simulink model "Rail_SetPointCor"  (R2016b)
settings: configuration reference "CodeGenConfigSet" (kept outside this file)
values from neighbouring files (symbols this model uses):
  Rail_facSetPointAPSCor_CUR = Calibration.Parameter    [init_Rail_SetPointCor.m]    (also in init_Rail_SetPointCor_SIL.m = Simulink.Parameter)
  Rail_facSetPointAPSCor_CURX = Calibration.Parameter    [init_Rail_SetPointCor.m]    (also in init_Rail_SetPointCor_SIL.m = Simulink.Parameter)
  Rail_facSetPointATSCor_CUR = Calibration.Parameter    [init_Rail_SetPointCor.m]    (also in init_Rail_SetPointCor_SIL.m = Simulink.Parameter)
  Rail_facSetPointATSCor_CURX = Calibration.Parameter    [init_Rail_SetPointCor.m]    (also in init_Rail_SetPointCor_SIL.m = Simulink.Parameter)
  Rail_facSetPointETSCor_CUR = Calibration.Parameter    [init_Rail_SetPointCor.m]    (also in init_Rail_SetPointCor_SIL.m = Simulink.Parameter)
  Rail_facSetPointETSCor_CURX = Calibration.Parameter    [init_Rail_SetPointCor.m]    (also in init_Rail_SetPointCor_SIL.m = Simulink.Parameter)
  Rail_pSetPointAPSCor_MAP = Calibration.Parameter    [init_Rail_SetPointCor.m]    (also in init_Rail_SetPointCor_SIL.m = Simulink.Parameter)
  Rail_pSetPointAPSCor_MAPX = Calibration.Parameter    [init_Rail_SetPointCor.m]    (also in init_Rail_SetPointCor_SIL.m = Simulink.Parameter)
  Rail_pSetPointAPSCor_MAPY = Calibration.Parameter    [init_Rail_SetPointCor.m]    (also in init_Rail_SetPointCor_SIL.m = Simulink.Parameter)
  Rail_pSetPointATSCor_MAP = Calibration.Parameter    [init_Rail_SetPointCor.m]    (also in init_Rail_SetPointCor_SIL.m = Simulink.Parameter)
  Rail_pSetPointATSCor_MAPX = Calibration.Parameter    [init_Rail_SetPointCor.m]    (also in init_Rail_SetPointCor_SIL.m = Simulink.Parameter)
  Rail_pSetPointATSCor_MAPY = Calibration.Parameter    [init_Rail_SetPointCor.m]    (also in init_Rail_SetPointCor_SIL.m = Simulink.Parameter)
  Rail_pSetPointETSCor_MAP = Calibration.Parameter    [init_Rail_SetPointCor.m]    (also in init_Rail_SetPointCor_SIL.m = Simulink.Parameter)
  Rail_pSetPointETSCor_MAPX = Calibration.Parameter    [init_Rail_SetPointCor.m]    (also in init_Rail_SetPointCor_SIL.m = Simulink.Parameter)
  Rail_pSetPointETSCor_MAPY = Calibration.Parameter    [init_Rail_SetPointCor.m]    (also in init_Rail_SetPointCor_SIL.m = Simulink.Parameter)
settings Model: Creator=lenovo  LastModifiedBy=zhoutinglin
settings ConfigSetRef: SourceLocation=Base Workspace

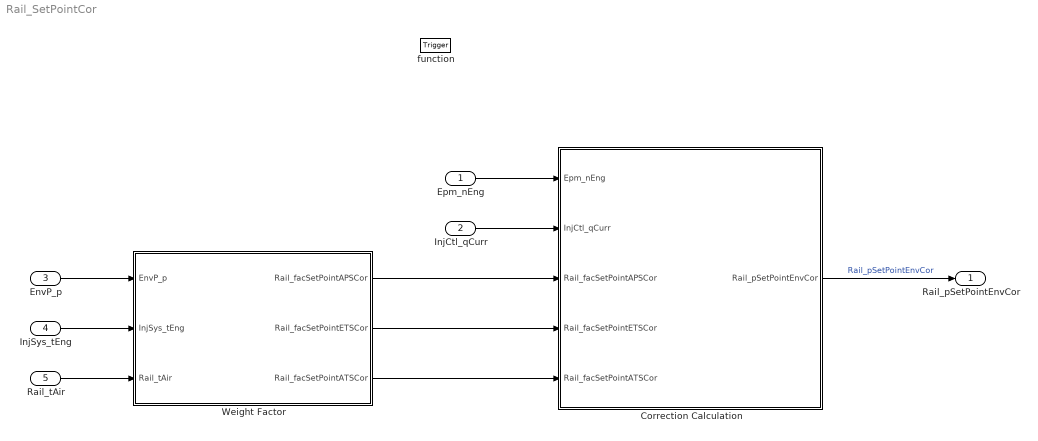
== system Rail_SetPointCor ==
  Epm_nEng : Inport  Tag=rpm  Description=Engine speed  OutMin=0  OutMax=6000  OutDataTypeStr=EngSpeed_rpm
  InjCtl_qCurr : Inport  Tag=mg/hub  Description=Torque generating engine fuel injection quantity  Port=2  OutMin=-319  OutMax=319  OutDataTypeStr=FuelMass_mg_hub
  EnvP_p : Inport  Tag=kPa  Description=Barometric pressure  Port=3  OutMin=0  OutMax=3276  OutDataTypeStr=AirPressure_kPa
  InjSys_tEng : Inport  Tag=deg  Description=Engine temperature selected for the injection system  Port=4  OutMin=-1000  OutMax=1000  OutDataTypeStr=Temp_deg
  Rail_tAir : Inport  Tag=deg  Description=Intake air temperature for the Rail subsystem  Port=5  OutMin=-1000  OutMax=1000  OutDataTypeStr=Temp_deg
  function : TriggerPort  TriggerType=function-call  VariantControl=Variant
  Correction Calculation : Subsystem
  Weight Factor : Subsystem
  Rail_pSetPointEnvCor : Outport  Tag=bar  Description=Corrected rail pressure setpoint based on environmental conditions (for present operation mode)  OutMin=-2500  OutMax=2500  OutDataTypeStr=RailPressure_bar
  wires:
  Correction Calculation/1(Rail_pSetPointEnvCor) -> Rail_pSetPointEnvCor/1  "Rail_pSetPointEnvCor"
  Epm_nEng/1 -> Correction Calculation/1(Epm_nEng)
  InjSys_tEng/1 -> Weight Factor/2(InjSys_tEng)
  EnvP_p/1 -> Weight Factor/1(EnvP_p)
  Rail_tAir/1 -> Weight Factor/3(Rail_tAir)
  InjCtl_qCurr/1 -> Correction Calculation/2(InjCtl_qCurr)
  Weight Factor/1(Rail_facSetPointAPSCor) -> Correction Calculation/3(Rail_facSetPointAPSCor)
  Weight Factor/2(Rail_facSetPointETSCor) -> Correction Calculation/4(Rail_facSetPointETSCor)
  Weight Factor/3(Rail_facSetPointATSCor) -> Correction Calculation/5(Rail_facSetPointATSCor)

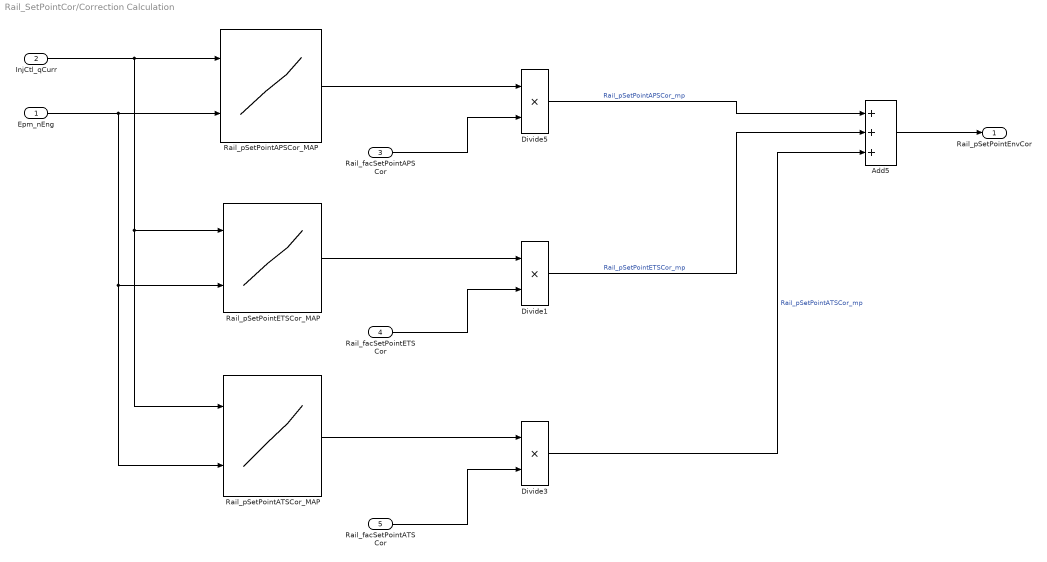
== system Rail_SetPointCor/Correction Calculation ==
  Epm_nEng : Inport
  InjCtl_qCurr : Inport  Port=2
  Rail_facSetPointAPSCor : Inport  Port=3
  Rail_facSetPointETSCor : Inport  Port=4
  Rail_facSetPointATSCor : Inport  Port=5
  Add5 : Sum  Inputs=+++  SaturateOnIntegerOverflow=on  InputSameDT=on
  Divide1 : Product  Inputs=**  OutDataTypeStr=RailPressure_bar  SaturateOnIntegerOverflow=on
  Divide3 : Product  Inputs=**  OutDataTypeStr=RailPressure_bar  SaturateOnIntegerOverflow=on
  Divide5 : Product  Inputs=**  OutDataTypeStr=RailPressure_bar  SaturateOnIntegerOverflow=on
  Rail_pSetPointAPSCor_MAP : Lookup_n-D  BreakpointsForDimension1=Rail_pSetPointAPSCor_MAPY  BreakpointsForDimension2=Rail_pSetPointAPSCor_MAPX  IndexSearchMethod=Linear search  BeginIndexSearchUsingPreviousIndexResult=on  Table=Rail_pSetPointAPSCor_MAP  ExtrapMethod=Clip  UseLastTableValue=on  InternalRulePriority=Speed  OutDataTypeStr=Inherit: Inherit via back propagation  SaturateOnIntegerOverflow=on
  Rail_pSetPointATSCor_MAP : Lookup_n-D  BreakpointsForDimension1=Rail_pSetPointATSCor_MAPY  BreakpointsForDimension2=Rail_pSetPointATSCor_MAPX  IndexSearchMethod=Linear search  BeginIndexSearchUsingPreviousIndexResult=on  Table=Rail_pSetPointATSCor_MAP  ExtrapMethod=Clip  UseLastTableValue=on  InternalRulePriority=Speed  OutDataTypeStr=Inherit: Inherit via back propagation  SaturateOnIntegerOverflow=on
  Rail_pSetPointETSCor_MAP : Lookup_n-D  BreakpointsForDimension1=Rail_pSetPointETSCor_MAPY  BreakpointsForDimension2=Rail_pSetPointETSCor_MAPX  IndexSearchMethod=Linear search  BeginIndexSearchUsingPreviousIndexResult=on  Table=Rail_pSetPointETSCor_MAP  ExtrapMethod=Clip  UseLastTableValue=on  InternalRulePriority=Speed  OutDataTypeStr=Inherit: Inherit via back propagation  SaturateOnIntegerOverflow=on
  Rail_pSetPointEnvCor : Outport
  wires:
  Rail_pSetPointATSCor_MAP/1 -> Divide3/1
  Rail_pSetPointETSCor_MAP/1 -> Divide1/1
  Add5/1 -> Rail_pSetPointEnvCor/1
  Divide3/1 -> Add5/3  "Rail_pSetPointATSCor_mp"
  Rail_facSetPointATSCor/1 -> Divide3/2
  Divide1/1 -> Add5/2  "Rail_pSetPointETSCor_mp"
  Rail_facSetPointETSCor/1 -> Divide1/2
  Divide5/1 -> Add5/1  "Rail_pSetPointAPSCor_mp"
  Rail_facSetPointAPSCor/1 -> Divide5/2
  Epm_nEng/1 -> Rail_pSetPointAPSCor_MAP/2, Rail_pSetPointETSCor_MAP/2, Rail_pSetPointATSCor_MAP/2
  InjCtl_qCurr/1 -> Rail_pSetPointAPSCor_MAP/1, Rail_pSetPointETSCor_MAP/1, Rail_pSetPointATSCor_MAP/1
  Rail_pSetPointAPSCor_MAP/1 -> Divide5/1

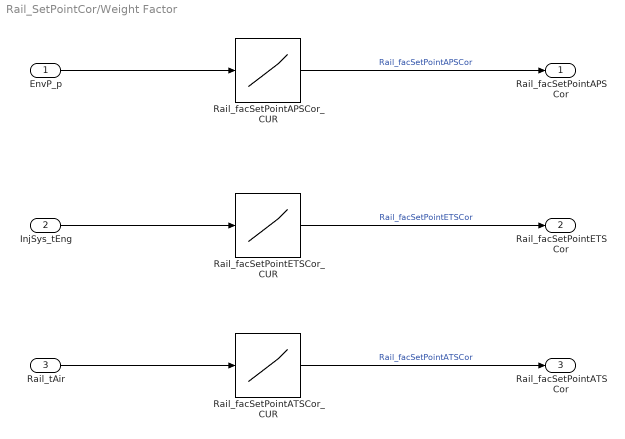
== system Rail_SetPointCor/Weight Factor ==
  EnvP_p : Inport
  InjSys_tEng : Inport  Port=2
  Rail_tAir : Inport  Port=3
  Rail_facSetPointAPSCor_CUR : Lookup_n-D  NumberOfTableDimensions=1  BreakpointsForDimension1=Rail_facSetPointAPSCor_CURX  IndexSearchMethod=Linear search  BeginIndexSearchUsingPreviousIndexResult=on  Table=Rail_facSetPointAPSCor_CUR  ExtrapMethod=Clip  UseLastTableValue=on  InternalRulePriority=Speed  OutDataTypeStr=Inherit: Inherit via back propagation  SaturateOnIntegerOverflow=on
  Rail_facSetPointATSCor_CUR : Lookup_n-D  NumberOfTableDimensions=1  BreakpointsForDimension1=Rail_facSetPointATSCor_CURX  IndexSearchMethod=Linear search  BeginIndexSearchUsingPreviousIndexResult=on  Table=Rail_facSetPointATSCor_CUR  ExtrapMethod=Clip  UseLastTableValue=on  InternalRulePriority=Speed  OutDataTypeStr=Inherit: Inherit via back propagation  SaturateOnIntegerOverflow=on
  Rail_facSetPointETSCor_CUR : Lookup_n-D  NumberOfTableDimensions=1  BreakpointsForDimension1=Rail_facSetPointETSCor_CURX  IndexSearchMethod=Linear search  BeginIndexSearchUsingPreviousIndexResult=on  Table=Rail_facSetPointETSCor_CUR  ExtrapMethod=Clip  UseLastTableValue=on  InternalRulePriority=Speed  OutDataTypeStr=Inherit: Inherit via back propagation  SaturateOnIntegerOverflow=on
  Rail_facSetPointAPSCor : Outport
  Rail_facSetPointETSCor : Outport  Port=2
  Rail_facSetPointATSCor : Outport  Port=3
  wires:
  Rail_facSetPointATSCor_CUR/1 -> Rail_facSetPointATSCor/1  "Rail_facSetPointATSCor"
  Rail_facSetPointETSCor_CUR/1 -> Rail_facSetPointETSCor/1  "Rail_facSetPointETSCor"
  Rail_facSetPointAPSCor_CUR/1 -> Rail_facSetPointAPSCor/1  "Rail_facSetPointAPSCor"
  EnvP_p/1 -> Rail_facSetPointAPSCor_CUR/1
  Rail_tAir/1 -> Rail_facSetPointATSCor_CUR/1
  InjSys_tEng/1 -> Rail_facSetPointETSCor_CUR/1
